simulink model "FOC_BLDC_HIL"  (R2021a)
settings: Solver=FixedStepDiscrete  StartTime=0.0  StopTime=2  RelTol=1e-3  EnableMultiTasking=on
undefined symbols (not defined in the file): DiscIntNeverNeededParam, Init_angle, J, Kawspeed, Ke, Kspeed, Lsx, Lsy, negVid, negVTm, oversampling, p, posVid, posVTm, Psim, Rs, T_load, Ts, ts_FPGA_clk, ts_FPGA_mdl, Ts_svpwm, Tsp, Vdc, Viq, VTm
libraries: simulink x93, hdlsllib x23, slrealtimeloglib x3
(part 4 of 4)

== system FOC_BLDC_HIL/Field Oriented Control/Current Controller/d//q controller/id controller ==
  id_error : Inport
  ed : Inport  Port=2
  "  " : Gain  Gain=100
  Abs : Abs  ZeroCross=off
  Discrete-Time Integrator : DiscreteIntegrator  SampleTime=Ts  LimitOutput=on  UpperSaturationLimit=48  LowerSaturationLimit=-48  ICPrevOutput=DiscIntNeverNeededParam  ICPrevScaledInput=DiscIntNeverNeededParam
  PID constant : Gain  Gain=0.01
  Product : Product
  Relay : Relay  OnOutputValue=0  OffOutputValue=1  ZeroCross=off
  Saturation : Saturate  UpperLimit=48  LowerLimit=-48  ZeroCross=off
  Sum : Sum  Inputs=+++
  Sum1 : Sum  Inputs=-+
  vd : Outport  VectorParamsAs1DForOutWhenUnconnected=off
  wires:
  "  "/1 -> Discrete-Time Integrator/1
  Sum/1 -> Sum1/2, Saturation/1
  Saturation/1 -> Sum1/1, vd/1
  Sum1/1 -> Abs/1
  Product/1 -> "  "/1
  Abs/1 -> Relay/1
  Relay/1 -> Product/1
  Discrete-Time Integrator/1 -> Sum/1
  PID constant/1 -> Sum/2, Product/2
  id_error/1 -> PID constant/1
  ed/1 -> Sum/3

== system FOC_BLDC_HIL/Field Oriented Control/Current Controller/d//q controller/iq controller ==
  iq_error : Inport
  eq : Inport  Port=2
  "  " : Gain  Gain=100
  Abs : Abs  ZeroCross=off
  Discrete-Time Integrator : DiscreteIntegrator  SampleTime=Ts  LimitOutput=on  UpperSaturationLimit=48  LowerSaturationLimit=-48  ICPrevOutput=DiscIntNeverNeededParam  ICPrevScaledInput=DiscIntNeverNeededParam
  PID constatn : Gain  Gain=0.01
  Product : Product
  Relay : Relay  OnOutputValue=0  OffOutputValue=1  ZeroCross=off
  Saturation : Saturate  UpperLimit=48  LowerLimit=-48  ZeroCross=off
  Sum : Sum  Inputs=+++
  Sum1 : Sum  Inputs=-+
  vq : Outport  VectorParamsAs1DForOutWhenUnconnected=off
  wires:
  PID constatn/1 -> Product/2, Sum/2
  Discrete-Time Integrator/1 -> Sum/1
  Relay/1 -> Product/1
  Abs/1 -> Relay/1
  Product/1 -> "  "/1
  Sum1/1 -> Abs/1
  Saturation/1 -> vq/1, Sum1/1
  Sum/1 -> Saturation/1, Sum1/2
  "  "/1 -> Discrete-Time Integrator/1
  iq_error/1 -> PID constatn/1
  eq/1 -> Sum/3

== system FOC_BLDC_HIL/Field Oriented Control/Speed Controller/Speed controller/Current reference generator ==
  T* : Inport
  Compare To Zero : simulink/Logic and Bit Operations/Compare To Zero  relop=<  OutDataTypeStr=boolean
  Mux : Mux  Inputs=2
  Switch : Switch  Criteria=u2 > Threshold
  id*neg : Lookup_n-D  NumberOfTableDimensions=1  BreakpointsForDimension1=negVTm  Table=negVid  ExtrapMethod=Clip  UseLastTableValue=on  InternalRulePriority=Speed  RndMeth=Simplest  InputSameDT=on
  id*pos : Lookup_n-D  NumberOfTableDimensions=1  BreakpointsForDimension1=posVTm  Table=posVid  ExtrapMethod=Clip  UseLastTableValue=on  InternalRulePriority=Speed  RndMeth=Simplest  InputSameDT=on
  iq* : Lookup_n-D  NumberOfTableDimensions=1  BreakpointsForDimension1=VTm  Table=Viq  ExtrapMethod=Clip  UseLastTableValue=on  InternalRulePriority=Speed  RndMeth=Simplest  InputSameDT=on
  idq_ref : Outport  VectorParamsAs1DForOutWhenUnconnected=off
  wires:
  Mux/1 -> idq_ref/1
  id*pos/1 -> Switch/3
  T*/1 -> id*neg/1, Compare To Zero/1, id*pos/1, iq*/1
  Switch/1 -> Mux/1
  iq*/1 -> Mux/2
  Compare To Zero/1 -> Switch/2
  id*neg/1 -> Switch/1

== system FOC_BLDC_HIL/Field Oriented Control/Speed Controller/Speed controller/Torque calculation ==
  idq_ref : Inport
  (p/2)*(3/2) : Gain  Gain=3*p/2
  Add : Sum
  Demux : Demux  Outputs=2
  Lsx-Lsy : Gain  Gain=Lsx-Lsy
  Product : Product
  Psim : Constant  Value=Psim  OutDataTypeStr=single
  Tmax : Outport  VectorParamsAs1DForOutWhenUnconnected=off
  wires:
  idq_ref/1 -> Demux/1
  (p/2)*(3/2)/1 -> Tmax/1
  Product/1 -> (p/2)*(3/2)/1
  Demux/2 -> Product/2
  Demux/1 -> Lsx-Lsy/1
  Psim/1 -> Add/1
  Lsx-Lsy/1 -> Add/2
  Add/1 -> Product/1

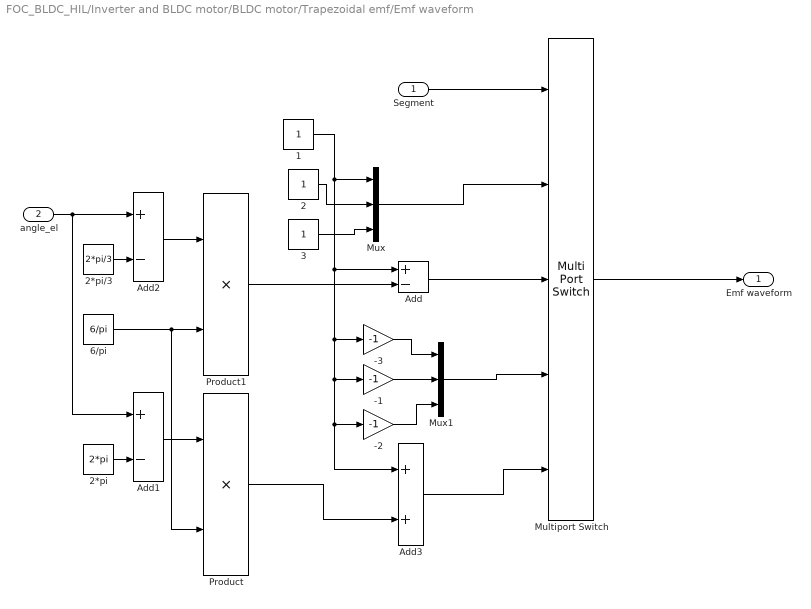
== system FOC_BLDC_HIL/Inverter and BLDC motor/BLDC motor/Trapezoidal emf/Emf waveform ==
  Segment : Inport
  angle_el : Inport  Port=2
  -1 : Gain  Gain=-1  OutDataTypeStr=single
  -2 : Gain  Gain=-1  OutDataTypeStr=single
  -3 : Gain  Gain=-1  OutDataTypeStr=single
  1 : Constant  OutDataTypeStr=single  SampleTime=-1
  2 : Constant  OutDataTypeStr=single  SampleTime=-1
  2*pi : Constant  Value=2*pi  OutDataTypeStr=single  SampleTime=-1
  2*pi/3 : Constant  Value=2*pi/3  OutDataTypeStr=single  SampleTime=-1
  3 : Constant  OutDataTypeStr=single  SampleTime=-1
  6/pi : Constant  Value=6/pi  OutDataTypeStr=single  SampleTime=-1
  Add : Sum  Inputs=+-  OutDataTypeStr=single
  Add1 : Sum  Inputs=+-
  Add2 : Sum  Inputs=+-  OutDataTypeStr=single
  Add3 : Sum  OutDataTypeStr=single
  Multiport Switch : MultiPortSwitch  Inputs=4  OutDataTypeStr=single  InputSameDT=on
  Mux : Mux  Inputs=3
  Mux1 : Mux  Inputs=3
  Product : Product  OutDataTypeStr=single
  Product1 : Product  OutDataTypeStr=single
  Emf waveform : Outport  VectorParamsAs1DForOutWhenUnconnected=off
  wires:
  Add2/1 -> Product1/1
  Product/1 -> Add3/2
  6/pi/1 -> Product1/2, Product/2
  2*pi/3/1 -> Add2/2
  Product1/1 -> Add/2
  Add1/1 -> Product/1
  2*pi/1 -> Add1/2
  angle_el/1 -> Add2/1, Add1/1
  Segment/1 -> Multiport Switch/1
  Multiport Switch/1 -> Emf waveform/1
  Add3/1 -> Multiport Switch/5
  Add/1 -> Multiport Switch/3
  3/1 -> Mux/3
  2/1 -> Mux/2
  -3/1 -> Mux1/1
  -1/1 -> Mux1/2
  -2/1 -> Mux1/3
  Mux1/1 -> Multiport Switch/4
  1/1 -> Mux/1, -3/1, -2/1, Add3/1, -1/1, Add/1
  Mux/1 -> Multiport Switch/2

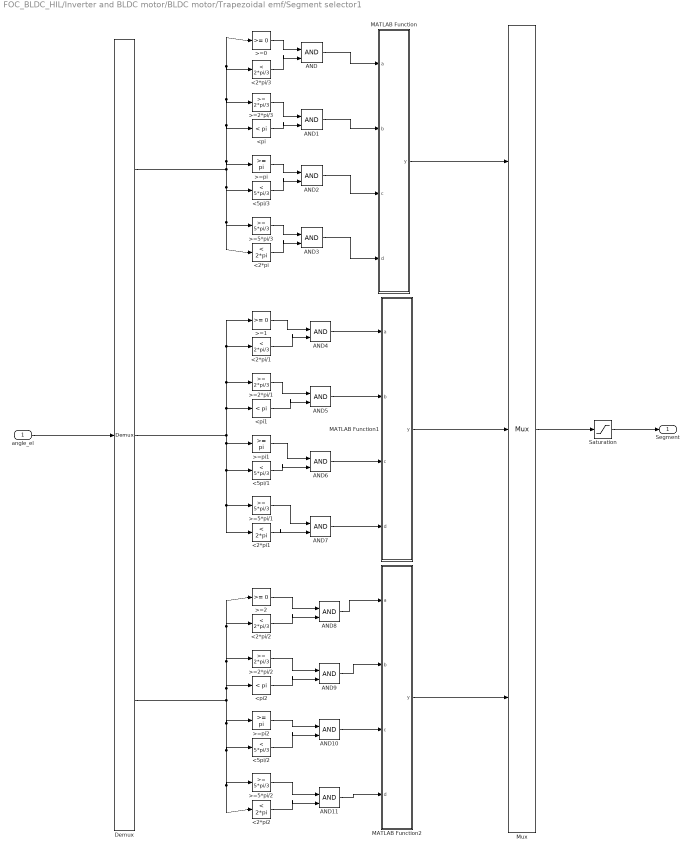
== system FOC_BLDC_HIL/Inverter and BLDC motor/BLDC motor/Trapezoidal emf/Segment selector1 ==
  angle_el : Inport
  <2*pi : simulink/Logic and Bit Operations/Compare To Constant  relop=<  const=2*pi  OutDataTypeStr=boolean  ZeroCross=off
  <2*pi/1 : simulink/Logic and Bit Operations/Compare To Constant  relop=<  const=2*pi/3  OutDataTypeStr=boolean  ZeroCross=off
  <2*pi/2 : simulink/Logic and Bit Operations/Compare To Constant  relop=<  const=2*pi/3  OutDataTypeStr=boolean  ZeroCross=off
  <2*pi/3 : simulink/Logic and Bit Operations/Compare To Constant  relop=<  const=2*pi/3  OutDataTypeStr=boolean  ZeroCross=off
  <2*pi1 : simulink/Logic and Bit Operations/Compare To Constant  relop=<  const=2*pi  OutDataTypeStr=boolean  ZeroCross=off
  <2*pi2 : simulink/Logic and Bit Operations/Compare To Constant  relop=<  const=2*pi  OutDataTypeStr=boolean  ZeroCross=off
  <5pi/1 : simulink/Logic and Bit Operations/Compare To Constant  relop=<  const=5*pi/3  OutDataTypeStr=boolean  ZeroCross=off
  <5pi/2 : simulink/Logic and Bit Operations/Compare To Constant  relop=<  const=5*pi/3  OutDataTypeStr=boolean  ZeroCross=off
  <5pi/3 : simulink/Logic and Bit Operations/Compare To Constant  relop=<  const=5*pi/3  OutDataTypeStr=boolean  ZeroCross=off
  <pi : simulink/Logic and Bit Operations/Compare To Constant  relop=<  const=pi  OutDataTypeStr=boolean  ZeroCross=off
  <pi1 : simulink/Logic and Bit Operations/Compare To Constant  relop=<  const=pi  OutDataTypeStr=boolean  ZeroCross=off
  <pi2 : simulink/Logic and Bit Operations/Compare To Constant  relop=<  const=pi  OutDataTypeStr=boolean  ZeroCross=off
  >=0 : simulink/Logic and Bit Operations/Compare To Constant  relop=>=  const=0  OutDataTypeStr=boolean  ZeroCross=off
  >=1 : simulink/Logic and Bit Operations/Compare To Constant  relop=>=  const=0  OutDataTypeStr=boolean  ZeroCross=off
  >=2 : simulink/Logic and Bit Operations/Compare To Constant  relop=>=  const=0  OutDataTypeStr=boolean  ZeroCross=off
  >=2*pi/1 : simulink/Logic and Bit Operations/Compare To Constant  relop=>=  const=2*pi/3  OutDataTypeStr=boolean  ZeroCross=off
  >=2*pi/2 : simulink/Logic and Bit Operations/Compare To Constant  relop=>=  const=2*pi/3  OutDataTypeStr=boolean  ZeroCross=off
  >=2*pi/3 : simulink/Logic and Bit Operations/Compare To Constant  relop=>=  const=2*pi/3  OutDataTypeStr=boolean  ZeroCross=off
  >=5*pi/1 : simulink/Logic and Bit Operations/Compare To Constant  relop=>=  const=5*pi/3  OutDataTypeStr=boolean  ZeroCross=off
  >=5*pi/2 : simulink/Logic and Bit Operations/Compare To Constant  relop=>=  const=5*pi/3  OutDataTypeStr=boolean  ZeroCross=off
  >=5*pi/3 : simulink/Logic and Bit Operations/Compare To Constant  relop=>=  const=5*pi/3  OutDataTypeStr=boolean  ZeroCross=off
  >=pi : simulink/Logic and Bit Operations/Compare To Constant  relop=>=  const=pi  OutDataTypeStr=boolean  ZeroCross=off
  >=pi1 : simulink/Logic and Bit Operations/Compare To Constant  relop=>=  const=pi  OutDataTypeStr=boolean  ZeroCross=off
  >=pi2 : simulink/Logic and Bit Operations/Compare To Constant  relop=>=  const=pi  OutDataTypeStr=boolean  ZeroCross=off
  AND{,1..11} (12 alike) : Logic  IconShape=distinctive  AllPortsSameDT=off  OutDataTypeStr=boolean
  Demux : Demux  Outputs=3
  MATLAB Function : MATLAB Function  TreatAsAtomicUnit=on
  MATLAB Function1 : MATLAB Function  TreatAsAtomicUnit=on
  MATLAB Function2 : MATLAB Function  TreatAsAtomicUnit=on
  Mux : Mux  Inputs=3
  Saturation : Saturate  UpperLimit=4  LowerLimit=1
  Segment : Outport  VectorParamsAs1DForOutWhenUnconnected=off
  wires:
  Demux/1 -> >=5*pi/3/1, <2*pi/1, <5pi/3/1, >=0/1, <2*pi/3/1, >=2*pi/3/1, <pi/1, >=pi/1
  <pi/1 -> AND1/2
  >=0/1 -> AND/1
  AND2/1 -> MATLAB Function/3(c)
  AND1/1 -> MATLAB Function/2(b)
  AND3/1 -> MATLAB Function/4(d)
  <2*pi/1 -> AND3/2
  >=5*pi/3/1 -> AND3/1
  >=2*pi/3/1 -> AND1/1
  <5pi/3/1 -> AND2/2
  <2*pi/3/1 -> AND/2
  >=pi/1 -> AND2/1
  AND/1 -> MATLAB Function/1(a)
  Saturation/1 -> Segment/1
  >=2*pi/1/1 -> AND5/1
  >=5*pi/1/1 -> AND7/1
  >=1/1 -> AND4/1
  >=pi1/1 -> AND6/1
  <pi1/1 -> AND5/2
  <2*pi/1/1 -> AND4/2
  <2*pi1/1 -> AND7/2
  Demux/2 -> >=5*pi/1/1, <2*pi1/1, <5pi/1/1, >=pi1/1, >=1/1, <2*pi/1/1, >=2*pi/1/1, <pi1/1
  <5pi/1/1 -> AND6/2
  >=2*pi/2/1 -> AND9/1
  >=5*pi/2/1 -> AND11/1
  >=2/1 -> AND8/1
  >=pi2/1 -> AND10/1
  <pi2/1 -> AND9/2
  <2*pi/2/1 -> AND8/2
  <2*pi2/1 -> AND11/2
  Demux/3 -> >=5*pi/2/1, <2*pi2/1, <5pi/2/1, >=pi2/1, >=2/1, <2*pi/2/1, >=2*pi/2/1, <pi2/1
  <5pi/2/1 -> AND10/2
  angle_el/1 -> Demux/1
  Mux/1 -> Saturation/1
  AND5/1 -> MATLAB Function1/2(b)
  AND7/1 -> MATLAB Function1/4(d)
  AND4/1 -> MATLAB Function1/1(a)
  AND6/1 -> MATLAB Function1/3(c)
  AND9/1 -> MATLAB Function2/2(b)
  AND11/1 -> MATLAB Function2/4(d)
  AND8/1 -> MATLAB Function2/1(a)
  AND10/1 -> MATLAB Function2/3(c)
  MATLAB Function1/1(y) -> Mux/2
  MATLAB Function/1(y) -> Mux/1
  MATLAB Function2/1(y) -> Mux/3

== system FOC_BLDC_HIL/Inverter and BLDC motor/BLDC motor/Trapezoidal emf/abc -> d//q ==
  eabc : Inport
  Sin : Inport  Port=2
  Cos : Inport  Port=3
  Demux : Demux  Outputs=3
  Gain : Gain  Gain=sqrt(3/2)
  Gain1 : Gain  Gain=sqrt(1/2)
  Gain2 : Gain  Gain=-1  OutDataTypeStr=single
  Mux2 : Mux  Inputs=2
  Product{,1..3} (4 alike) : Product
  Subtract : Sum  Inputs=+-
  Subtract1 : Sum
  Sum : Sum  Inputs=+|-
  edq : Outport  VectorParamsAs1DForOutWhenUnconnected=off
  wires:
  eabc/1 -> Demux/1
  Demux/1 -> Gain/1
  Demux/2 -> Sum/1
  Demux/3 -> Sum/2
  Gain/1 -> Product2/1, Product/1  "Alpha"
  Mux2/1 -> edq/1
  Sum/1 -> Gain1/1
  Cos/1 -> Product3/2, Product/2
  Gain1/1 -> Product3/1, Product1/1  "Beta"
  Sin/1 -> Gain2/1
  Product/1 -> Subtract/1
  Product1/1 -> Subtract/2
  Subtract/1 -> Mux2/1
  Product2/1 -> Subtract1/1
  Product3/1 -> Subtract1/2
  Subtract1/1 -> Mux2/2
  Gain2/1 -> Product1/2, Product2/2

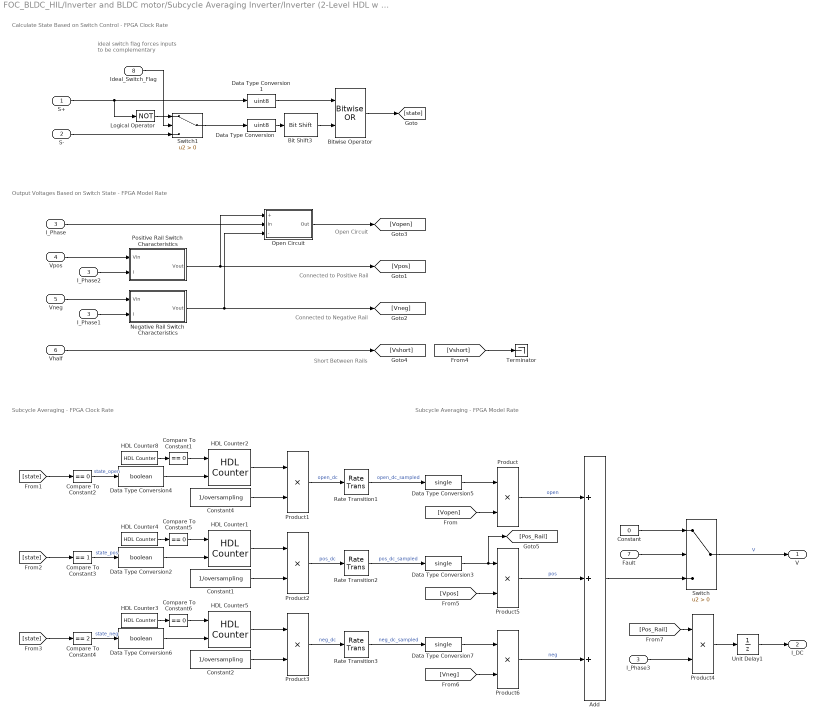
== system FOC_BLDC_HIL/Inverter and BLDC motor/Subcycle Averaging Inverter/Inverter (2-Level HDL w faults)/Calculate Phase Voltage ==
  note: Subcycle Averaging - FPGA Clock Rate
  note: ideal switch flag forces
      | inputs to be complementary
  note: Open Circuit
  note: Connected to Positive Rail
  note: Connected to Negative Rail
  note: Short Between Rails
  note: Subcycle Averaging - FPGA Model Rate
  note: Output Voltages Based on Switch State - FPGA Model Rate
  note: Calculate State Based on Switch Control - FPGA Clock Rate
  S+ : Inport
  S- : Inport  Port=2
  I_Phase : Inport  Port=3
  Vpos : Inport  Port=4
  Vneg : Inport  Port=5
  Vhalf : Inport  Port=6
  Fault : Inport  Port=7
  Ideal_Switch_Flag : Inport  Port=8
  Add : Sum  Inputs=+++
  Bit Shift3 : hdlsllib/Logic and Bit Operations/Bit Shift  mode=Shift Left Logical  N=1
  Bitwise Operator : simulink/Logic and Bit Operations/Bitwise Operator  logicop=OR  UseBitMask=off  NumInputPorts=2  BitMask=bin2dec('11011001')  BitMaskRealWorld=Stored Integer
  Compare To Constant{1..2,5..6} (4 alike) : simulink/Logic and Bit Operations/Compare To Constant  relop===  const=0  OutDataTypeStr=boolean
  Compare To Constant3 : simulink/Logic and Bit Operations/Compare To Constant  relop===  const=1  OutDataTypeStr=boolean
  Compare To Constant4 : simulink/Logic and Bit Operations/Compare To Constant  relop===  const=2  OutDataTypeStr=boolean
  Constant : Constant  Value=0  OutDataTypeStr=single  SampleTime=ts_FPGA_mdl
  Constant1 : Constant  Value=1/oversampling  OutDataTypeStr=fixdt(0,18,18)  SampleTime=ts_FPGA_clk
  Constant2 : Constant  Value=1/oversampling  OutDataTypeStr=fixdt(0,18,18)  SampleTime=ts_FPGA_clk
  Constant4 : Constant  Value=1/oversampling  OutDataTypeStr=fixdt(0,18,18)  SampleTime=ts_FPGA_clk
  Data Type Conversion : DataTypeConversion  OutDataTypeStr=uint8
  Data Type Conversion1 : DataTypeConversion  OutDataTypeStr=uint8
  Data Type Conversion2 : DataTypeConversion  OutDataTypeStr=boolean
  Data Type Conversion3 : DataTypeConversion  OutDataTypeStr=single
  Data Type Conversion4 : DataTypeConversion  OutDataTypeStr=boolean
  Data Type Conversion5 : DataTypeConversion  OutDataTypeStr=single
  Data Type Conversion6 : DataTypeConversion  OutDataTypeStr=boolean
  Data Type Conversion7 : DataTypeConversion  OutDataTypeStr=single
  HDL Counter1 : hdlsllib/Sources/HDL Counter  CountType=Count limited  CountInit=1  CountStep=1  CountMax=oversampling  CountFromType=Initial value  CountFrom=1  CountResetPort=on  CountLoadPort=off  CountEnbPort=on  CountDirPort=off  CountHitOutputPort=off  CountDataType=Unsigned  CountWordLen=8  CountFracLen=0  CountSampTime=1
  HDL Counter2 : hdlsllib/Sources/HDL Counter  CountType=Count limited  CountInit=1  CountStep=1  CountMax=oversampling  CountFromType=Initial value  CountFrom=1  CountResetPort=on  CountLoadPort=off  CountEnbPort=on  CountDirPort=off  CountHitOutputPort=off  CountDataType=Unsigned  CountWordLen=8  CountFracLen=0  CountSampTime=1
  HDL Counter3 : hdlsllib/Sources/HDL Counter  CountType=Count limited  CountInit=0  CountStep=1  CountMax=oversampling-1  CountFromType=Initial value  CountFrom=0  CountResetPort=off  CountLoadPort=off  CountEnbPort=off  CountDirPort=off  CountHitOutputPort=off  CountDataType=Unsigned  CountWordLen=8  CountFracLen=0  CountSampTime=ts_FPGA_clk
  HDL Counter4 : hdlsllib/Sources/HDL Counter  CountType=Count limited  CountInit=0  CountStep=1  CountMax=oversampling-1  CountFromType=Initial value  CountFrom=0  CountResetPort=off  CountLoadPort=off  CountEnbPort=off  CountDirPort=off  CountHitOutputPort=off  CountDataType=Unsigned  CountWordLen=8  CountFracLen=0  CountSampTime=ts_FPGA_clk
  HDL Counter5 : hdlsllib/Sources/HDL Counter  CountType=Count limited  CountInit=1  CountStep=1  CountMax=oversampling  CountFromType=Initial value  CountFrom=1  CountResetPort=on  CountLoadPort=off  CountEnbPort=on  CountDirPort=off  CountHitOutputPort=off  CountDataType=Unsigned  CountWordLen=8  CountFracLen=0  CountSampTime=1
  HDL Counter8 : hdlsllib/Sources/HDL Counter  CountType=Count limited  CountInit=0  CountStep=1  CountMax=oversampling-1  CountFromType=Initial value  CountFrom=0  CountResetPort=off  CountLoadPort=off  CountEnbPort=off  CountDirPort=off  CountHitOutputPort=off  CountDataType=Unsigned  CountWordLen=8  CountFracLen=0  CountSampTime=ts_FPGA_clk
  I_Phase1 : InportShadow  Port=3
  I_Phase2 : InportShadow  Port=3
  I_Phase3 : InportShadow  Port=3
  Logical Operator : Logic  Operator=NOT  AllPortsSameDT=off  OutDataTypeStr=boolean
  Negative Rail Switch Characteristics : Subsystem
  Open Circuit : Subsystem
  Positive Rail Switch Characteristics : Subsystem
  Product{,1..6} (7 alike) : Product
  Rate Transition1 : RateTransition  OutPortSampleTime=1e-6
  Rate Transition2 : RateTransition  OutPortSampleTime=1e-6
  Rate Transition3 : RateTransition  OutPortSampleTime=1e-6
  Switch : Switch  Criteria=u2 > Threshold
  Switch1 : Switch  Criteria=u2 > Threshold
  Terminator : Terminator
  Unit Delay1 : UnitDelay  SampleTime=-1  HasFrameUpgradeWarning=on
  V : Outport  VectorParamsAs1DForOutWhenUnconnected=off
  I_DC : Outport  Port=2  VectorParamsAs1DForOutWhenUnconnected=off
  wires:
  Switch/1 -> V/1  "V"
  Bit Shift3/1 -> Bitwise Operator/2
  Vpos/1 -> Positive Rail Switch Characteristics/1(Vin)
  Vhalf/1 -> [Vshort]
  Open Circuit/1(Out) -> [Vopen]
  Data Type Conversion/1 -> Bit Shift3/1
  Data Type Conversion1/1 -> Bitwise Operator/1
  Vneg/1 -> Negative Rail Switch Characteristics/1(Vin)
  S-/1 -> Switch1/3
  I_Phase/1 -> Open Circuit/2(In)
  Fault/1 -> Switch/2
  Constant/1 -> Switch/1
  Negative Rail Switch Characteristics/1(Vout) -> [Vneg], Open Circuit/3(-)
  Positive Rail Switch Characteristics/1(Vout) -> [Vpos], Open Circuit/1(+)
  I_Phase2/1 -> Positive Rail Switch Characteristics/2(I)
  I_Phase1/1 -> Negative Rail Switch Characteristics/2(I)
  Ideal_Switch_Flag/1 -> Switch1/2
  Logical Operator/1 -> Switch1/1
  Switch1/1 -> Data Type Conversion/1
  Rate Transition1/1 -> Data Type Conversion5/1  "open_dc_sampled"
  HDL Counter8/1 -> Compare To Constant1/1
  Constant4/1 -> Product1/2
  Data Type Conversion4/1 -> HDL Counter2/2
  Compare To Constant1/1 -> HDL Counter2/1
  Product1/1 -> Rate Transition1/1  "open_dc"
  HDL Counter2/1 -> Product1/1
  S+/1 -> Logical Operator/1, Data Type Conversion1/1
  Bitwise Operator/1 -> [state]
  [state] -> Compare To Constant3/1
  [state] -> Compare To Constant2/1
  [state] -> Compare To Constant4/1
  HDL Counter1/1 -> Product2/1
  Product2/1 -> Rate Transition2/1  "pos_dc"
  Compare To Constant5/1 -> HDL Counter1/1
  Data Type Conversion2/1 -> HDL Counter1/2
  Constant1/1 -> Product2/2
  HDL Counter4/1 -> Compare To Constant5/1
  Rate Transition2/1 -> Data Type Conversion3/1  "pos_dc_sampled"
  Rate Transition3/1 -> Data Type Conversion7/1  "neg_dc_sampled"
  HDL Counter3/1 -> Compare To Constant6/1
  Constant2/1 -> Product3/2
  Data Type Conversion6/1 -> HDL Counter5/2
  Compare To Constant6/1 -> HDL Counter5/1
  Product3/1 -> Rate Transition3/1  "neg_dc"
  HDL Counter5/1 -> Product3/1
  Compare To Constant4/1 -> Data Type Conversion6/1  "state_neg"
  Compare To Constant3/1 -> Data Type Conversion2/1  "state_pos"
  Compare To Constant2/1 -> Data Type Conversion4/1  "state_open"
  Add/1 -> Switch/3
  Data Type Conversion5/1 -> Product/1
  [Vopen] -> Product/2
  Data Type Conversion3/1 -> [Pos_Rail], Product5/1
  [Vpos] -> Product5/2
  Data Type Conversion7/1 -> Product6/1
  [Vneg] -> Product6/2
  Product/1 -> Add/1  "open"
  Product5/1 -> Add/2  "pos"
  Product6/1 -> Add/3  "neg"
  [Vshort] -> Terminator/1
  Product4/1 -> Unit Delay1/1
  I_Phase3/1 -> Product4/2
  [Pos_Rail] -> Product4/1
  Unit Delay1/1 -> I_DC/1

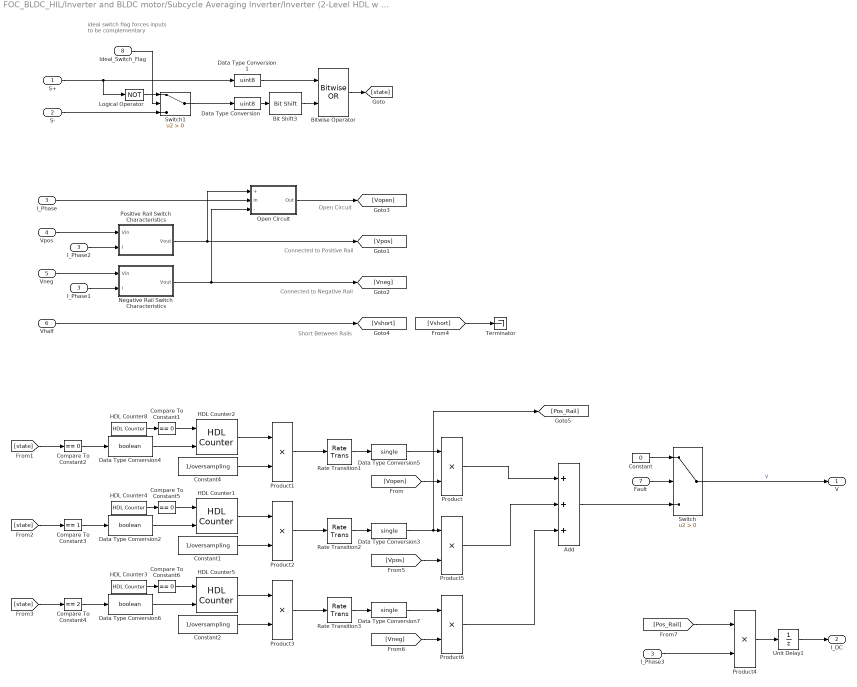
== system FOC_BLDC_HIL/Inverter and BLDC motor/Subcycle Averaging Inverter/Inverter (2-Level HDL w faults)/Calculate Phase Voltage1 ==
  note: Short Between Rails
  note: Connected to Negative Rail
  note: Connected to Positive Rail
  note: Open Circuit
  note: ideal switch flag forces
      | inputs to be complementary
  S+ : Inport
  S- : Inport  Port=2
  I_Phase : Inport  Port=3
  Vpos : Inport  Port=4
  Vneg : Inport  Port=5
  Vhalf : Inport  Port=6
  Fault : Inport  Port=7
  Ideal_Switch_Flag : Inport  Port=8
  Add : Sum  Inputs=+++
  Bit Shift3 : hdlsllib/Logic and Bit Operations/Bit Shift  mode=Shift Left Logical  N=1
  Bitwise Operator : simulink/Logic and Bit Operations/Bitwise Operator  logicop=OR  UseBitMask=off  NumInputPorts=2  BitMask=bin2dec('11011001')  BitMaskRealWorld=Stored Integer
  Compare To Constant{1..2,5..6} (4 alike) : simulink/Logic and Bit Operations/Compare To Constant  relop===  const=0  OutDataTypeStr=boolean
  Compare To Constant3 : simulink/Logic and Bit Operations/Compare To Constant  relop===  const=1  OutDataTypeStr=boolean
  Compare To Constant4 : simulink/Logic and Bit Operations/Compare To Constant  relop===  const=2  OutDataTypeStr=boolean
  Constant : Constant  Value=0  OutDataTypeStr=single  SampleTime=ts_FPGA_mdl
  Constant1 : Constant  Value=1/oversampling  OutDataTypeStr=fixdt(0,18,18)  SampleTime=ts_FPGA_clk
  Constant2 : Constant  Value=1/oversampling  OutDataTypeStr=fixdt(0,18,18)  SampleTime=ts_FPGA_clk
  Constant4 : Constant  Value=1/oversampling  OutDataTypeStr=fixdt(0,18,18)  SampleTime=ts_FPGA_clk
  Data Type Conversion : DataTypeConversion  OutDataTypeStr=uint8
  Data Type Conversion1 : DataTypeConversion  OutDataTypeStr=uint8
  Data Type Conversion2 : DataTypeConversion  OutDataTypeStr=boolean
  Data Type Conversion3 : DataTypeConversion  OutDataTypeStr=single
  Data Type Conversion4 : DataTypeConversion  OutDataTypeStr=boolean
  Data Type Conversion5 : DataTypeConversion  OutDataTypeStr=single
  Data Type Conversion6 : DataTypeConversion  OutDataTypeStr=boolean
  Data Type Conversion7 : DataTypeConversion  OutDataTypeStr=single
  HDL Counter1 : hdlsllib/Sources/HDL Counter  CountType=Count limited  CountInit=1  CountStep=1  CountMax=oversampling  CountFromType=Initial value  CountFrom=1  CountResetPort=on  CountLoadPort=off  CountEnbPort=on  CountDirPort=off  CountHitOutputPort=off  CountDataType=Unsigned  CountWordLen=8  CountFracLen=0  CountSampTime=1
  HDL Counter2 : hdlsllib/Sources/HDL Counter  CountType=Count limited  CountInit=1  CountStep=1  CountMax=oversampling  CountFromType=Initial value  CountFrom=1  CountResetPort=on  CountLoadPort=off  CountEnbPort=on  CountDirPort=off  CountHitOutputPort=off  CountDataType=Unsigned  CountWordLen=8  CountFracLen=0  CountSampTime=1
  HDL Counter3 : hdlsllib/Sources/HDL Counter  CountType=Count limited  CountInit=0  CountStep=1  CountMax=oversampling-1  CountFromType=Initial value  CountFrom=0  CountResetPort=off  CountLoadPort=off  CountEnbPort=off  CountDirPort=off  CountHitOutputPort=off  CountDataType=Unsigned  CountWordLen=8  CountFracLen=0  CountSampTime=ts_FPGA_clk
  HDL Counter4 : hdlsllib/Sources/HDL Counter  CountType=Count limited  CountInit=0  CountStep=1  CountMax=oversampling-1  CountFromType=Initial value  CountFrom=0  CountResetPort=off  CountLoadPort=off  CountEnbPort=off  CountDirPort=off  CountHitOutputPort=off  CountDataType=Unsigned  CountWordLen=8  CountFracLen=0  CountSampTime=ts_FPGA_clk
  HDL Counter5 : hdlsllib/Sources/HDL Counter  CountType=Count limited  CountInit=1  CountStep=1  CountMax=oversampling  CountFromType=Initial value  CountFrom=1  CountResetPort=on  CountLoadPort=off  CountEnbPort=on  CountDirPort=off  CountHitOutputPort=off  CountDataType=Unsigned  CountWordLen=8  CountFracLen=0  CountSampTime=1
  HDL Counter8 : hdlsllib/Sources/HDL Counter  CountType=Count limited  CountInit=0  CountStep=1  CountMax=oversampling-1  CountFromType=Initial value  CountFrom=0  CountResetPort=off  CountLoadPort=off  CountEnbPort=off  CountDirPort=off  CountHitOutputPort=off  CountDataType=Unsigned  CountWordLen=8  CountFracLen=0  CountSampTime=ts_FPGA_clk
  I_Phase1 : InportShadow  Port=3
  I_Phase2 : InportShadow  Port=3
  I_Phase3 : InportShadow  Port=3
  Logical Operator : Logic  Operator=NOT  AllPortsSameDT=off  OutDataTypeStr=boolean
  Negative Rail Switch Characteristics : Subsystem
  Open Circuit : Subsystem
  Positive Rail Switch Characteristics : Subsystem
  Product{,1..6} (7 alike) : Product
  Rate Transition1 : RateTransition  OutPortSampleTime=1e-6
  Rate Transition2 : RateTransition  OutPortSampleTime=1e-6
  Rate Transition3 : RateTransition  OutPortSampleTime=1e-6
  Switch : Switch  Criteria=u2 > Threshold
  Switch1 : Switch  Criteria=u2 > Threshold
  Terminator : Terminator
  Unit Delay1 : UnitDelay  SampleTime=-1  HasFrameUpgradeWarning=on
  V : Outport  VectorParamsAs1DForOutWhenUnconnected=off
  I_DC : Outport  Port=2  VectorParamsAs1DForOutWhenUnconnected=off
  wires:
  Unit Delay1/1 -> I_DC/1
  [Pos_Rail] -> Product4/1
  I_Phase3/1 -> Product4/2
  Product4/1 -> Unit Delay1/1
  [Vshort] -> Terminator/1
  Product6/1 -> Add/3
  Product5/1 -> Add/2
  Product/1 -> Add/1
  [Vneg] -> Product6/2
  Data Type Conversion7/1 -> Product6/1
  [Vpos] -> Product5/2
  Data Type Conversion3/1 -> Product5/1, [Pos_Rail]
  [Vopen] -> Product/2
  Data Type Conversion5/1 -> Product/1
  Add/1 -> Switch/3
  Compare To Constant2/1 -> Data Type Conversion4/1
  Compare To Constant3/1 -> Data Type Conversion2/1
  Compare To Constant4/1 -> Data Type Conversion6/1
  HDL Counter5/1 -> Product3/1
  Product3/1 -> Rate Transition3/1
  Compare To Constant6/1 -> HDL Counter5/1
  Data Type Conversion6/1 -> HDL Counter5/2
  Constant2/1 -> Product3/2
  HDL Counter3/1 -> Compare To Constant6/1
  Rate Transition3/1 -> Data Type Conversion7/1
  Rate Transition2/1 -> Data Type Conversion3/1
  HDL Counter4/1 -> Compare To Constant5/1
  Constant1/1 -> Product2/2
  Data Type Conversion2/1 -> HDL Counter1/2
  Compare To Constant5/1 -> HDL Counter1/1
  Product2/1 -> Rate Transition2/1
  HDL Counter1/1 -> Product2/1
  [state] -> Compare To Constant4/1
  [state] -> Compare To Constant2/1
  [state] -> Compare To Constant3/1
  Bitwise Operator/1 -> [state]
  S+/1 -> Data Type Conversion1/1, Logical Operator/1
  HDL Counter2/1 -> Product1/1
  Product1/1 -> Rate Transition1/1
  Compare To Constant1/1 -> HDL Counter2/1
  Data Type Conversion4/1 -> HDL Counter2/2
  Constant4/1 -> Product1/2
  HDL Counter8/1 -> Compare To Constant1/1
  Rate Transition1/1 -> Data Type Conversion5/1
  Switch1/1 -> Data Type Conversion/1
  Logical Operator/1 -> Switch1/1
  Ideal_Switch_Flag/1 -> Switch1/2
  I_Phase1/1 -> Negative Rail Switch Characteristics/2(I)
  I_Phase2/1 -> Positive Rail Switch Characteristics/2(I)
  Positive Rail Switch Characteristics/1(Vout) -> Open Circuit/1(+), [Vpos]
  Negative Rail Switch Characteristics/1(Vout) -> Open Circuit/3(-), [Vneg]
  Constant/1 -> Switch/1
  Fault/1 -> Switch/2
  I_Phase/1 -> Open Circuit/2(In)
  S-/1 -> Switch1/3
  Vneg/1 -> Negative Rail Switch Characteristics/1(Vin)
  Data Type Conversion1/1 -> Bitwise Operator/1
  Data Type Conversion/1 -> Bit Shift3/1
  Open Circuit/1(Out) -> [Vopen]
  Vhalf/1 -> [Vshort]
  Vpos/1 -> Positive Rail Switch Characteristics/1(Vin)
  Bit Shift3/1 -> Bitwise Operator/2
  Switch/1 -> V/1  "V"

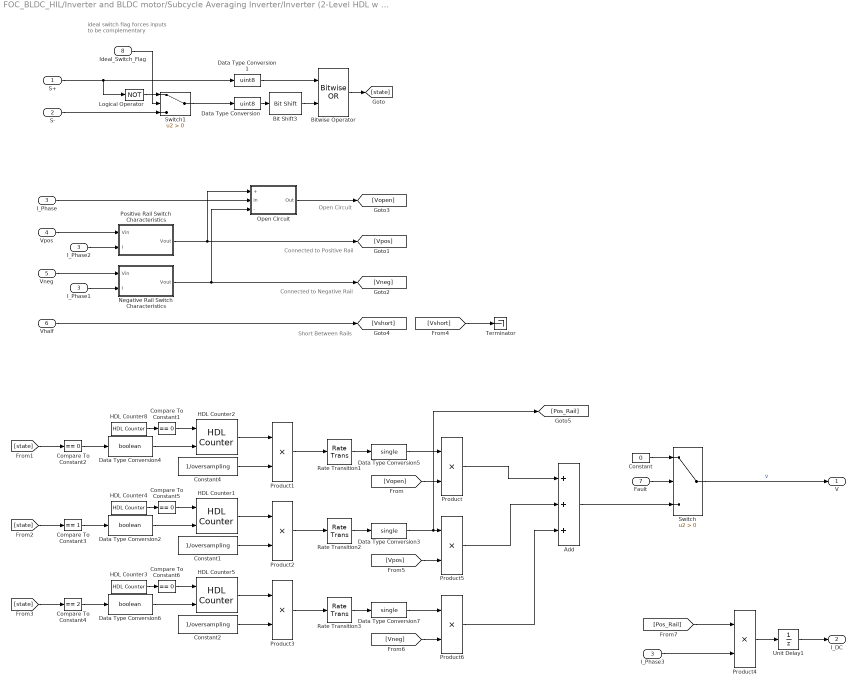
== system FOC_BLDC_HIL/Inverter and BLDC motor/Subcycle Averaging Inverter/Inverter (2-Level HDL w faults)/Calculate Phase Voltage2 ==
  note: ideal switch flag forces
      | inputs to be complementary
  note: Open Circuit
  note: Connected to Positive Rail
  note: Connected to Negative Rail
  note: Short Between Rails
  S+ : Inport
  S- : Inport  Port=2
  I_Phase : Inport  Port=3
  Vpos : Inport  Port=4
  Vneg : Inport  Port=5
  Vhalf : Inport  Port=6
  Fault : Inport  Port=7
  Ideal_Switch_Flag : Inport  Port=8
  Add : Sum  Inputs=+++
  Bit Shift3 : hdlsllib/Logic and Bit Operations/Bit Shift  mode=Shift Left Logical  N=1
  Bitwise Operator : simulink/Logic and Bit Operations/Bitwise Operator  logicop=OR  UseBitMask=off  NumInputPorts=2  BitMask=bin2dec('11011001')  BitMaskRealWorld=Stored Integer
  Compare To Constant{1..2,5..6} (4 alike) : simulink/Logic and Bit Operations/Compare To Constant  relop===  const=0  OutDataTypeStr=boolean
  Compare To Constant3 : simulink/Logic and Bit Operations/Compare To Constant  relop===  const=1  OutDataTypeStr=boolean
  Compare To Constant4 : simulink/Logic and Bit Operations/Compare To Constant  relop===  const=2  OutDataTypeStr=boolean
  Constant : Constant  Value=0  OutDataTypeStr=single  SampleTime=ts_FPGA_mdl
  Constant1 : Constant  Value=1/oversampling  OutDataTypeStr=fixdt(0,18,18)  SampleTime=ts_FPGA_clk
  Constant2 : Constant  Value=1/oversampling  OutDataTypeStr=fixdt(0,18,18)  SampleTime=ts_FPGA_clk
  Constant4 : Constant  Value=1/oversampling  OutDataTypeStr=fixdt(0,18,18)  SampleTime=ts_FPGA_clk
  Data Type Conversion : DataTypeConversion  OutDataTypeStr=uint8
  Data Type Conversion1 : DataTypeConversion  OutDataTypeStr=uint8
  Data Type Conversion2 : DataTypeConversion  OutDataTypeStr=boolean
  Data Type Conversion3 : DataTypeConversion  OutDataTypeStr=single
  Data Type Conversion4 : DataTypeConversion  OutDataTypeStr=boolean
  Data Type Conversion5 : DataTypeConversion  OutDataTypeStr=single
  Data Type Conversion6 : DataTypeConversion  OutDataTypeStr=boolean
  Data Type Conversion7 : DataTypeConversion  OutDataTypeStr=single
  HDL Counter1 : hdlsllib/Sources/HDL Counter  CountType=Count limited  CountInit=1  CountStep=1  CountMax=oversampling  CountFromType=Initial value  CountFrom=1  CountResetPort=on  CountLoadPort=off  CountEnbPort=on  CountDirPort=off  CountHitOutputPort=off  CountDataType=Unsigned  CountWordLen=8  CountFracLen=0  CountSampTime=1
  HDL Counter2 : hdlsllib/Sources/HDL Counter  CountType=Count limited  CountInit=1  CountStep=1  CountMax=oversampling  CountFromType=Initial value  CountFrom=1  CountResetPort=on  CountLoadPort=off  CountEnbPort=on  CountDirPort=off  CountHitOutputPort=off  CountDataType=Unsigned  CountWordLen=8  CountFracLen=0  CountSampTime=1
  HDL Counter3 : hdlsllib/Sources/HDL Counter  CountType=Count limited  CountInit=0  CountStep=1  CountMax=oversampling-1  CountFromType=Initial value  CountFrom=0  CountResetPort=off  CountLoadPort=off  CountEnbPort=off  CountDirPort=off  CountHitOutputPort=off  CountDataType=Unsigned  CountWordLen=8  CountFracLen=0  CountSampTime=ts_FPGA_clk
  HDL Counter4 : hdlsllib/Sources/HDL Counter  CountType=Count limited  CountInit=0  CountStep=1  CountMax=oversampling-1  CountFromType=Initial value  CountFrom=0  CountResetPort=off  CountLoadPort=off  CountEnbPort=off  CountDirPort=off  CountHitOutputPort=off  CountDataType=Unsigned  CountWordLen=8  CountFracLen=0  CountSampTime=ts_FPGA_clk
  HDL Counter5 : hdlsllib/Sources/HDL Counter  CountType=Count limited  CountInit=1  CountStep=1  CountMax=oversampling  CountFromType=Initial value  CountFrom=1  CountResetPort=on  CountLoadPort=off  CountEnbPort=on  CountDirPort=off  CountHitOutputPort=off  CountDataType=Unsigned  CountWordLen=8  CountFracLen=0  CountSampTime=1
  HDL Counter8 : hdlsllib/Sources/HDL Counter  CountType=Count limited  CountInit=0  CountStep=1  CountMax=oversampling-1  CountFromType=Initial value  CountFrom=0  CountResetPort=off  CountLoadPort=off  CountEnbPort=off  CountDirPort=off  CountHitOutputPort=off  CountDataType=Unsigned  CountWordLen=8  CountFracLen=0  CountSampTime=ts_FPGA_clk
  I_Phase1 : InportShadow  Port=3
  I_Phase2 : InportShadow  Port=3
  I_Phase3 : InportShadow  Port=3
  Logical Operator : Logic  Operator=NOT  AllPortsSameDT=off  OutDataTypeStr=boolean
  Negative Rail Switch Characteristics : Subsystem
  Open Circuit : Subsystem
  Positive Rail Switch Characteristics : Subsystem
  Product{,1..6} (7 alike) : Product
  Rate Transition1 : RateTransition  OutPortSampleTime=1e-6
  Rate Transition2 : RateTransition  OutPortSampleTime=1e-6
  Rate Transition3 : RateTransition  OutPortSampleTime=1e-6
  Switch : Switch  Criteria=u2 > Threshold
  Switch1 : Switch  Criteria=u2 > Threshold
  Terminator : Terminator
  Unit Delay1 : UnitDelay  SampleTime=-1  HasFrameUpgradeWarning=on
  V : Outport  VectorParamsAs1DForOutWhenUnconnected=off
  I_DC : Outport  Port=2  VectorParamsAs1DForOutWhenUnconnected=off
  wires:
  Switch/1 -> V/1  "V"
  Bit Shift3/1 -> Bitwise Operator/2
  Vpos/1 -> Positive Rail Switch Characteristics/1(Vin)
  Vhalf/1 -> [Vshort]
  Open Circuit/1(Out) -> [Vopen]
  Data Type Conversion/1 -> Bit Shift3/1
  Data Type Conversion1/1 -> Bitwise Operator/1
  Vneg/1 -> Negative Rail Switch Characteristics/1(Vin)
  S-/1 -> Switch1/3
  I_Phase/1 -> Open Circuit/2(In)
  Fault/1 -> Switch/2
  Constant/1 -> Switch/1
  Negative Rail Switch Characteristics/1(Vout) -> [Vneg], Open Circuit/3(-)
  Positive Rail Switch Characteristics/1(Vout) -> [Vpos], Open Circuit/1(+)
  I_Phase2/1 -> Positive Rail Switch Characteristics/2(I)
  I_Phase1/1 -> Negative Rail Switch Characteristics/2(I)
  Ideal_Switch_Flag/1 -> Switch1/2
  Logical Operator/1 -> Switch1/1
  Switch1/1 -> Data Type Conversion/1
  Rate Transition1/1 -> Data Type Conversion5/1
  HDL Counter8/1 -> Compare To Constant1/1
  Constant4/1 -> Product1/2
  Data Type Conversion4/1 -> HDL Counter2/2
  Compare To Constant1/1 -> HDL Counter2/1
  Product1/1 -> Rate Transition1/1
  HDL Counter2/1 -> Product1/1
  S+/1 -> Logical Operator/1, Data Type Conversion1/1
  Bitwise Operator/1 -> [state]
  [state] -> Compare To Constant3/1
  [state] -> Compare To Constant2/1
  [state] -> Compare To Constant4/1
  HDL Counter1/1 -> Product2/1
  Product2/1 -> Rate Transition2/1
  Compare To Constant5/1 -> HDL Counter1/1
  Data Type Conversion2/1 -> HDL Counter1/2
  Constant1/1 -> Product2/2
  HDL Counter4/1 -> Compare To Constant5/1
  Rate Transition2/1 -> Data Type Conversion3/1
  Rate Transition3/1 -> Data Type Conversion7/1
  HDL Counter3/1 -> Compare To Constant6/1
  Constant2/1 -> Product3/2
  Data Type Conversion6/1 -> HDL Counter5/2
  Compare To Constant6/1 -> HDL Counter5/1
  Product3/1 -> Rate Transition3/1
  HDL Counter5/1 -> Product3/1
  Compare To Constant4/1 -> Data Type Conversion6/1
  Compare To Constant3/1 -> Data Type Conversion2/1
  Compare To Constant2/1 -> Data Type Conversion4/1
  Add/1 -> Switch/3
  Data Type Conversion5/1 -> Product/1
  [Vopen] -> Product/2
  Data Type Conversion3/1 -> [Pos_Rail], Product5/1
  [Vpos] -> Product5/2
  Data Type Conversion7/1 -> Product6/1
  [Vneg] -> Product6/2
  Product/1 -> Add/1
  Product5/1 -> Add/2
  Product6/1 -> Add/3
  [Vshort] -> Terminator/1
  Product4/1 -> Unit Delay1/1
  I_Phase3/1 -> Product4/2
  [Pos_Rail] -> Product4/1
  Unit Delay1/1 -> I_DC/1

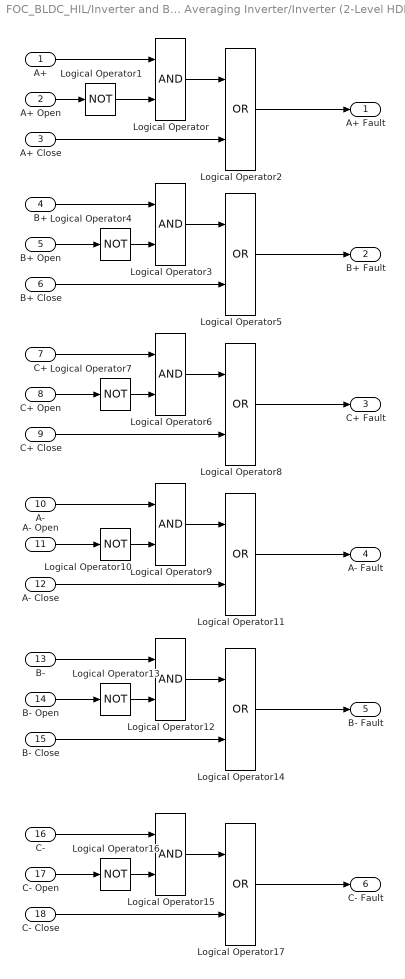
== system FOC_BLDC_HIL/Inverter and BLDC motor/Subcycle Averaging Inverter/Inverter (2-Level HDL w faults)/Incorporate Fault Signals ==
  A+ : Inport
  A+ Open : Inport  Port=2
  A+ Close : Inport  Port=3
  B+ : Inport  Port=4
  B+ Open : Inport  Port=5
  B+ Close : Inport  Port=6
  C+ : Inport  Port=7
  C+ Open : Inport  Port=8
  C+ Close : Inport  Port=9
  A- : Inport  Port=10
  A- Open : Inport  Port=11
  A- Close : Inport  Port=12
  B- : Inport  Port=13
  B- Open : Inport  Port=14
  B- Close : Inport  Port=15
  C- : Inport  Port=16
  C- Open : Inport  Port=17
  C- Close : Inport  Port=18
  Logical Operator{,3,6,9,12,15} (6 alike) : Logic  AllPortsSameDT=off  OutDataTypeStr=boolean
  Logical Operator{1,4,7,10,13,16} (6 alike) : Logic  Operator=NOT  AllPortsSameDT=off  OutDataTypeStr=boolean
  Logical Operator{2,5,8,11,14,17} (6 alike) : Logic  Operator=OR  AllPortsSameDT=off  OutDataTypeStr=boolean
  A+ Fault : Outport  VectorParamsAs1DForOutWhenUnconnected=off
  B+ Fault : Outport  Port=2  VectorParamsAs1DForOutWhenUnconnected=off
  C+ Fault : Outport  Port=3  VectorParamsAs1DForOutWhenUnconnected=off
  A- Fault : Outport  Port=4  VectorParamsAs1DForOutWhenUnconnected=off
  B- Fault : Outport  Port=5  VectorParamsAs1DForOutWhenUnconnected=off
  C- Fault : Outport  Port=6  VectorParamsAs1DForOutWhenUnconnected=off
  wires:
  Logical Operator1/1 -> Logical Operator/2
  A+ Open/1 -> Logical Operator1/1
  A+/1 -> Logical Operator/1
  A+ Close/1 -> Logical Operator2/2
  Logical Operator/1 -> Logical Operator2/1
  Logical Operator2/1 -> A+ Fault/1
  Logical Operator5/1 -> B+ Fault/1
  Logical Operator3/1 -> Logical Operator5/1
  B+ Close/1 -> Logical Operator5/2
  B+/1 -> Logical Operator3/1
  B+ Open/1 -> Logical Operator4/1
  Logical Operator4/1 -> Logical Operator3/2
  Logical Operator7/1 -> Logical Operator6/2
  C+/1 -> Logical Operator6/1
  C+ Close/1 -> Logical Operator8/2
  Logical Operator6/1 -> Logical Operator8/1
  Logical Operator8/1 -> C+ Fault/1
  Logical Operator11/1 -> A- Fault/1
  Logical Operator9/1 -> Logical Operator11/1
  A- Close/1 -> Logical Operator11/2
  A-/1 -> Logical Operator9/1
  Logical Operator10/1 -> Logical Operator9/2
  Logical Operator14/1 -> B- Fault/1
  Logical Operator12/1 -> Logical Operator14/1
  Logical Operator13/1 -> Logical Operator12/2
  B-/1 -> Logical Operator12/1
  B- Close/1 -> Logical Operator14/2
  Logical Operator17/1 -> C- Fault/1
  Logical Operator15/1 -> Logical Operator17/1
  Logical Operator16/1 -> Logical Operator15/2
  C-/1 -> Logical Operator15/1
  C- Close/1 -> Logical Operator17/2
  A- Open/1 -> Logical Operator10/1
  B- Open/1 -> Logical Operator13/1
  C- Open/1 -> Logical Operator16/1
  C+ Open/1 -> Logical Operator7/1

== system FOC_BLDC_HIL/Inverter and BLDC motor/Subcycle Averaging Inverter/Inverter (2-Level HDL w faults)/Vll_calculate ==
  V1 : Inport
  V2 : Inport  Port=2
  Fault : Inport  Port=3
  Constant : Constant  Value=0  OutDataTypeStr=single  SampleTime=-1
  Subtract2 : Sum  Inputs=+-
  Switch : Switch  Criteria=u2 > Threshold
  V12 : Outport  VectorParamsAs1DForOutWhenUnconnected=off
  wires:
  V2/1 -> Subtract2/2
  V1/1 -> Subtract2/1
  Subtract2/1 -> Switch/3  "V"
  Fault/1 -> Switch/2
  Switch/1 -> V12/1  "V"
  Constant/1 -> Switch/1

== system FOC_BLDC_HIL/Inverter and BLDC motor/Subcycle Averaging Inverter/Inverter (2-Level HDL w faults)/Vll_calculate1 ==
  V1 : Inport
  V2 : Inport  Port=2
  Fault : Inport  Port=3
  Constant : Constant  Value=0  OutDataTypeStr=single  SampleTime=-1
  Subtract2 : Sum  Inputs=+-
  Switch : Switch  Criteria=u2 > Threshold
  V12 : Outport  VectorParamsAs1DForOutWhenUnconnected=off
  wires:
  Constant/1 -> Switch/1
  Switch/1 -> V12/1  "V"
  Fault/1 -> Switch/2
  Subtract2/1 -> Switch/3  "V"
  V1/1 -> Subtract2/1
  V2/1 -> Subtract2/2

== system FOC_BLDC_HIL/Inverter and BLDC motor/Subcycle Averaging Inverter/Inverter (2-Level HDL w faults)/Vll_calculate2 ==
  V1 : Inport
  V2 : Inport  Port=2
  Fault : Inport  Port=3
  Constant : Constant  Value=0  OutDataTypeStr=single  SampleTime=-1
  Subtract2 : Sum  Inputs=+-
  Switch : Switch  Criteria=u2 > Threshold
  V12 : Outport  VectorParamsAs1DForOutWhenUnconnected=off
  wires:
  V2/1 -> Subtract2/2
  V1/1 -> Subtract2/1
  Subtract2/1 -> Switch/3  "V"
  Fault/1 -> Switch/2
  Switch/1 -> V12/1  "V"
  Constant/1 -> Switch/1

== system FOC_BLDC_HIL/Inverter and BLDC motor/Subcycle Averaging Inverter/Inverter (2-Level HDL w faults)/Calculate Phase Voltage/Negative Rail Switch Characteristics ==
  Vin : Inport
  I : Inport  Port=2
  Compare To Zero : simulink/Logic and Bit Operations/Compare To Zero  relop=>=  OutDataTypeStr=boolean
  Constant : Constant  Value=vfSwitch  OutDataTypeStr=single  SampleTime=ts_FPGA_mdl
  Constant1 : Constant  Value=vfDiode  OutDataTypeStr=single  SampleTime=ts_FPGA_mdl
  Gain : Gain  Gain=rSwitch
  Gain1 : Gain  Gain=rDiode
  I1 : InportShadow  Port=2
  I2 : InportShadow  Port=2
  Sum1 : Sum  Inputs=+-|
  Sum2 : Sum  Inputs=|--
  Sum3 : Sum  Inputs=++|
  Switch : Switch  Criteria=u2 > Threshold
  Unit Delay : UnitDelay  SampleTime=-1  HasFrameUpgradeWarning=on
  Vout : Outport  VectorParamsAs1DForOutWhenUnconnected=off
  wires:
  I/1 -> Gain/1
  Gain1/1 -> Sum2/1
  Sum3/1 -> Unit Delay/1
  Switch/1 -> Sum3/2
  I1/1 -> Compare To Zero/1
  Vin/1 -> Sum3/1
  Unit Delay/1 -> Vout/1
  Constant/1 -> Sum1/1
  I2/1 -> Gain1/1
  Sum1/1 -> Switch/3
  Gain/1 -> Sum1/2
  Sum2/1 -> Switch/1
  Constant1/1 -> Sum2/2
  Compare To Zero/1 -> Switch/2

== system FOC_BLDC_HIL/Inverter and BLDC motor/Subcycle Averaging Inverter/Inverter (2-Level HDL w faults)/Calculate Phase Voltage/Open Circuit ==
  + : Inport
  In : Inport  Port=2
  - : Inport  Port=3
  Gain : Gain  Gain=-rSnub
  Max : MinMax  Inputs=2
  Max1 : MinMax  Function=max  Inputs=2
  Unit Delay : UnitDelay  SampleTime=-1  HasFrameUpgradeWarning=on
  Out : Outport  VectorParamsAs1DForOutWhenUnconnected=off
  wires:
  -/1 -> Max1/2
  Max/1 -> Unit Delay/1
  +/1 -> Max/1
  Gain/1 -> Max1/1
  In/1 -> Gain/1
  Max1/1 -> Max/2
  Unit Delay/1 -> Out/1

== system FOC_BLDC_HIL/Inverter and BLDC motor/Subcycle Averaging Inverter/Inverter (2-Level HDL w faults)/Calculate Phase Voltage/Positive Rail Switch Characteristics ==
  Vin : Inport
  I : Inport  Port=2
  Compare To Zero : simulink/Logic and Bit Operations/Compare To Zero  relop=>=  OutDataTypeStr=boolean
  Constant : Constant  Value=vfSwitch  OutDataTypeStr=single  SampleTime=ts_FPGA_mdl
  Constant1 : Constant  Value=vfDiode  OutDataTypeStr=single  SampleTime=ts_FPGA_mdl
  Gain : Gain  Gain=rSwitch
  Gain1 : Gain  Gain=rDiode
  I1 : InportShadow  Port=2
  I2 : InportShadow  Port=2
  Sum1 : Sum  Inputs=-+|
  Sum2 : Sum  Inputs=|++
  Sum3 : Sum  Inputs=+-|
  Switch : Switch  Criteria=u2 > Threshold
  Unit Delay : UnitDelay  SampleTime=-1  HasFrameUpgradeWarning=on
  Vout : Outport  VectorParamsAs1DForOutWhenUnconnected=off
  wires:
  I/1 -> Gain/1
  Constant/1 -> Sum2/2
  Sum2/1 -> Switch/1
  Unit Delay/1 -> Vout/1
  Gain/1 -> Sum2/1
  Vin/1 -> Sum3/1
  I1/1 -> Compare To Zero/1
  Switch/1 -> Sum3/2
  Gain1/1 -> Sum1/2
  Constant1/1 -> Sum1/1
  I2/1 -> Gain1/1
  Sum1/1 -> Switch/3
  Sum3/1 -> Unit Delay/1
  Compare To Zero/1 -> Switch/2

== system FOC_BLDC_HIL/Inverter and BLDC motor/Subcycle Averaging Inverter/Inverter (2-Level HDL w faults)/Calculate Phase Voltage1/Negative Rail Switch Characteristics ==
  Vin : Inport
  I : Inport  Port=2
  Compare To Zero : simulink/Logic and Bit Operations/Compare To Zero  relop=>=  OutDataTypeStr=boolean
  Constant : Constant  Value=vfSwitch  OutDataTypeStr=single  SampleTime=ts_FPGA_mdl
  Constant1 : Constant  Value=vfDiode  OutDataTypeStr=single  SampleTime=ts_FPGA_mdl
  Gain : Gain  Gain=rSwitch
  Gain1 : Gain  Gain=rDiode
  I1 : InportShadow  Port=2
  I2 : InportShadow  Port=2
  Sum1 : Sum  Inputs=+-|
  Sum2 : Sum  Inputs=|--
  Sum3 : Sum  Inputs=++|
  Switch : Switch  Criteria=u2 > Threshold
  Unit Delay : UnitDelay  SampleTime=-1  HasFrameUpgradeWarning=on
  Vout : Outport  VectorParamsAs1DForOutWhenUnconnected=off
  wires:
  Compare To Zero/1 -> Switch/2
  Constant1/1 -> Sum2/2
  Sum2/1 -> Switch/1
  Gain/1 -> Sum1/2
  Sum1/1 -> Switch/3
  I2/1 -> Gain1/1
  Constant/1 -> Sum1/1
  Unit Delay/1 -> Vout/1
  Vin/1 -> Sum3/1
  I1/1 -> Compare To Zero/1
  Switch/1 -> Sum3/2
  Sum3/1 -> Unit Delay/1
  Gain1/1 -> Sum2/1
  I/1 -> Gain/1

== system FOC_BLDC_HIL/Inverter and BLDC motor/Subcycle Averaging Inverter/Inverter (2-Level HDL w faults)/Calculate Phase Voltage1/Open Circuit ==
  + : Inport
  In : Inport  Port=2
  - : Inport  Port=3
  Gain : Gain  Gain=-rSnub
  Max : MinMax  Inputs=2
  Max1 : MinMax  Function=max  Inputs=2
  Unit Delay : UnitDelay  SampleTime=-1  HasFrameUpgradeWarning=on
  Out : Outport  VectorParamsAs1DForOutWhenUnconnected=off
  wires:
  Unit Delay/1 -> Out/1
  Max1/1 -> Max/2
  In/1 -> Gain/1
  Gain/1 -> Max1/1
  +/1 -> Max/1
  Max/1 -> Unit Delay/1
  -/1 -> Max1/2

== system FOC_BLDC_HIL/Inverter and BLDC motor/Subcycle Averaging Inverter/Inverter (2-Level HDL w faults)/Calculate Phase Voltage1/Positive Rail Switch Characteristics ==
  Vin : Inport
  I : Inport  Port=2
  Compare To Zero : simulink/Logic and Bit Operations/Compare To Zero  relop=>=  OutDataTypeStr=boolean
  Constant : Constant  Value=vfSwitch  OutDataTypeStr=single  SampleTime=ts_FPGA_mdl
  Constant1 : Constant  Value=vfDiode  OutDataTypeStr=single  SampleTime=ts_FPGA_mdl
  Gain : Gain  Gain=rSwitch
  Gain1 : Gain  Gain=rDiode
  I1 : InportShadow  Port=2
  I2 : InportShadow  Port=2
  Sum1 : Sum  Inputs=-+|
  Sum2 : Sum  Inputs=|++
  Sum3 : Sum  Inputs=+-|
  Switch : Switch  Criteria=u2 > Threshold
  Unit Delay : UnitDelay  SampleTime=-1  HasFrameUpgradeWarning=on
  Vout : Outport  VectorParamsAs1DForOutWhenUnconnected=off
  wires:
  Compare To Zero/1 -> Switch/2
  Sum3/1 -> Unit Delay/1
  Sum1/1 -> Switch/3
  I2/1 -> Gain1/1
  Constant1/1 -> Sum1/1
  Gain1/1 -> Sum1/2
  Switch/1 -> Sum3/2
  I1/1 -> Compare To Zero/1
  Vin/1 -> Sum3/1
  Gain/1 -> Sum2/1
  Unit Delay/1 -> Vout/1
  Sum2/1 -> Switch/1
  Constant/1 -> Sum2/2
  I/1 -> Gain/1

== system FOC_BLDC_HIL/Inverter and BLDC motor/Subcycle Averaging Inverter/Inverter (2-Level HDL w faults)/Calculate Phase Voltage2/Negative Rail Switch Characteristics ==
  Vin : Inport
  I : Inport  Port=2
  Compare To Zero : simulink/Logic and Bit Operations/Compare To Zero  relop=>=  OutDataTypeStr=boolean
  Constant : Constant  Value=vfSwitch  OutDataTypeStr=single  SampleTime=ts_FPGA_mdl
  Constant1 : Constant  Value=vfDiode  OutDataTypeStr=single  SampleTime=ts_FPGA_mdl
  Gain : Gain  Gain=rSwitch
  Gain1 : Gain  Gain=rDiode
  I1 : InportShadow  Port=2
  I2 : InportShadow  Port=2
  Sum1 : Sum  Inputs=+-|
  Sum2 : Sum  Inputs=|--
  Sum3 : Sum  Inputs=++|
  Switch : Switch  Criteria=u2 > Threshold
  Unit Delay : UnitDelay  SampleTime=-1  HasFrameUpgradeWarning=on
  Vout : Outport  VectorParamsAs1DForOutWhenUnconnected=off
  wires:
  I/1 -> Gain/1
  Gain1/1 -> Sum2/1
  Sum3/1 -> Unit Delay/1
  Switch/1 -> Sum3/2
  I1/1 -> Compare To Zero/1
  Vin/1 -> Sum3/1
  Unit Delay/1 -> Vout/1
  Constant/1 -> Sum1/1
  I2/1 -> Gain1/1
  Sum1/1 -> Switch/3
  Gain/1 -> Sum1/2
  Sum2/1 -> Switch/1
  Constant1/1 -> Sum2/2
  Compare To Zero/1 -> Switch/2

== system FOC_BLDC_HIL/Inverter and BLDC motor/Subcycle Averaging Inverter/Inverter (2-Level HDL w faults)/Calculate Phase Voltage2/Open Circuit ==
  + : Inport
  In : Inport  Port=2
  - : Inport  Port=3
  Gain : Gain  Gain=-rSnub
  Max : MinMax  Inputs=2
  Max1 : MinMax  Function=max  Inputs=2
  Unit Delay : UnitDelay  SampleTime=-1  HasFrameUpgradeWarning=on
  Out : Outport  VectorParamsAs1DForOutWhenUnconnected=off
  wires:
  -/1 -> Max1/2
  Max/1 -> Unit Delay/1
  +/1 -> Max/1
  Gain/1 -> Max1/1
  In/1 -> Gain/1
  Max1/1 -> Max/2
  Unit Delay/1 -> Out/1

== system FOC_BLDC_HIL/Inverter and BLDC motor/Subcycle Averaging Inverter/Inverter (2-Level HDL w faults)/Calculate Phase Voltage2/Positive Rail Switch Characteristics ==
  Vin : Inport
  I : Inport  Port=2
  Compare To Zero : simulink/Logic and Bit Operations/Compare To Zero  relop=>=  OutDataTypeStr=boolean
  Constant : Constant  Value=vfSwitch  OutDataTypeStr=single  SampleTime=ts_FPGA_mdl
  Constant1 : Constant  Value=vfDiode  OutDataTypeStr=single  SampleTime=ts_FPGA_mdl
  Gain : Gain  Gain=rSwitch
  Gain1 : Gain  Gain=rDiode
  I1 : InportShadow  Port=2
  I2 : InportShadow  Port=2
  Sum1 : Sum  Inputs=-+|
  Sum2 : Sum  Inputs=|++
  Sum3 : Sum  Inputs=+-|
  Switch : Switch  Criteria=u2 > Threshold
  Unit Delay : UnitDelay  SampleTime=-1  HasFrameUpgradeWarning=on
  Vout : Outport  VectorParamsAs1DForOutWhenUnconnected=off
  wires:
  I/1 -> Gain/1
  Constant/1 -> Sum2/2
  Sum2/1 -> Switch/1
  Unit Delay/1 -> Vout/1
  Gain/1 -> Sum2/1
  Vin/1 -> Sum3/1
  I1/1 -> Compare To Zero/1
  Switch/1 -> Sum3/2
  Gain1/1 -> Sum1/2
  Constant1/1 -> Sum1/1
  I2/1 -> Gain1/1
  Sum1/1 -> Switch/3
  Sum3/1 -> Unit Delay/1
  Compare To Zero/1 -> Switch/2

== matlab function FOC_BLDC_HIL/Inverter and BLDC motor/BLDC motor/Trapezoidal emf/Segment selector1/MATLAB Function ==
  data: a input; y output; b input; c input; d input
function y = fcn(a,b,c,d)
if a==1
    y = fi(1,0,8,0);
elseif b==1
    y = fi(2,0,8,0);
elseif c==1
    y = fi(3,0,8,0);
elseif d==1
    y = fi(4,0,8,0);
else
    y = fi(0,0,8,0);
end

== matlab function FOC_BLDC_HIL/Inverter and BLDC motor/BLDC motor/Trapezoidal emf/Segment selector1/MATLAB Function1 ==
  data: a input; y output; b input; c input; d input
function y = fcn(a,b,c,d)
if a==1
    y = fi(1,0,8,0);
elseif b==1
    y = fi(2,0,8,0);
elseif c==1
    y = fi(3,0,8,0);
elseif d==1
    y = fi(4,0,8,0);
else
    y = fi(0,0,8,0);
end

== matlab function FOC_BLDC_HIL/Inverter and BLDC motor/BLDC motor/Trapezoidal emf/Segment selector1/MATLAB Function2 ==
  data: a input; y output; b input; c input; d input
function y = fcn(a,b,c,d)
if a==1
    y = fi(1,0,8,0);
elseif b==1
    y = fi(2,0,8,0);
elseif c==1
    y = fi(3,0,8,0);
elseif d==1
    y = fi(4,0,8,0);
else
    y = fi(0,0,8,0);
end
